simulink model "synchro_v3"  (R2020b)
settings: Solver=FixedStepAuto  StartTime=0.0  StopTime=2  FixedStep=Ts  RelTol=1e-3
values from neighbouring files (symbols this model uses):
  m = 5/100    (= 0.05)    [synchro_parameters_v1.m]
  Sbase = 1    [synchro_parameters_v1.m]
  Ts = 1/Fs    (= 0.0001)    [synchro_parameters_v1.m]
  Vbase = 1    [synchro_parameters_v1.m]
  w_droop = 10*2*pi    (= 62.8318530718)    [synchro_parameters_v1.m]
  w_pll = 10*2*pi    (= 62.8318530718)    [synchro_parameters_v1.m]
  w_tau = 1e3*2*pi    (= 6283.18530718)    [synchro_parameters_v1.m]
  Wbase = 2*pi*50    (= 314.159265359)    [synchro_parameters_v1.m]
  Ybase = 1/Zbase    (= 1)    [synchro_parameters_v1.m]
  Zbase = Vbase/Ibase    (= 1)    [synchro_parameters_v1.m]
undefined symbols (not defined in the file or in its folder): DiscIntNeverNeededParam
libraries: SimplexPS x69, powerlib x64
(part 2 of 2)

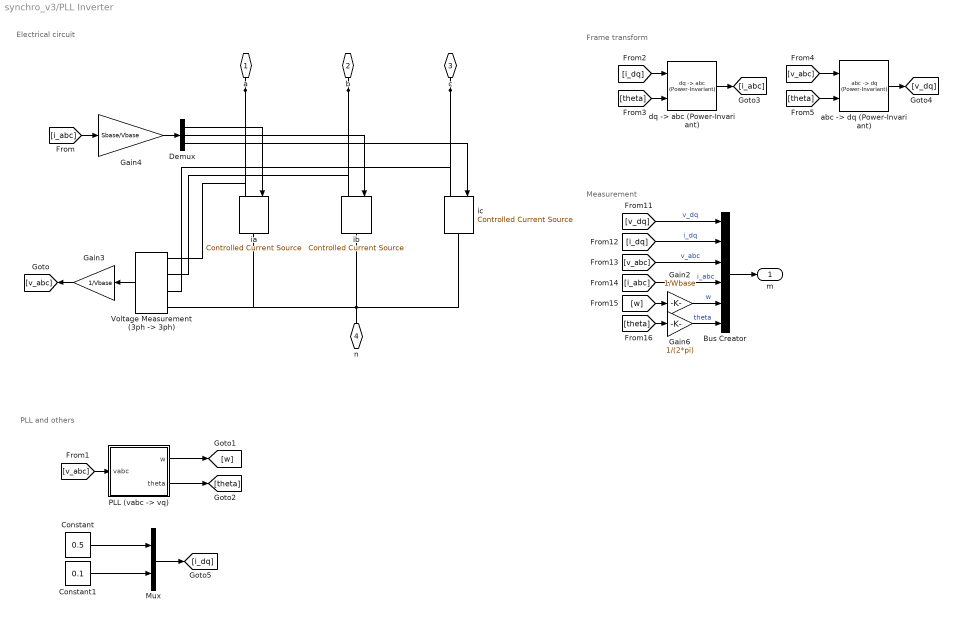
== system synchro_v3/PLL Inverter ==
  note: Measurement
  note: PLL and others
  note: Frame transform
  note: Electrical circuit
  Bus Creator : BusCreator  Inputs=6
  Constant : Constant  Value=0.5
  Constant1 : Constant  Value=0.1
  Demux : Demux  Outputs=3
  Gain2 : Gain  Gain=1/Wbase
  Gain3 : Gain  Gain=1/Vbase
  Gain4 : Gain  Gain=Sbase/Vbase
  Gain6 : Gain  Gain=1/(2*pi)
  Mux : Mux  Inputs=2
  "PLL (vabc -> vq)" : Subsystem  AncestorBlock=|  mask{Ts=Ts, Vbase=Vbase, Wbase=Wbase, w_pll=w_pll, w_tau=w_tau, theta0=0}
      | SimplexPS/PLL
      | (vabc -> vq)
      mask prompts: Ts "Ts (s), sampling period"; Vbase "Vbase (V), base voltage"; Wbase "Wbase (rad/s), base angular frequency"; w_pll "w_pll (rad/s), PLL bandwidth"; w_tau "w_tau (rad/s), low-pass filter bandwidth"; theta0 "theta0 (rad), initial angle"
  "Voltage Measurement (3ph -> 3ph)" : SimplexPS/Voltage Measurement (3ph -> 3ph)  SystemSampleTime=-1  VariantActivationTime=update diagram  Latency=0  AutoFrameSizeCalculation=off
      settings: SourceProductName=Simplex Power Systems
  "abc -> dq (Power-Invariant)" : SimplexPS/abc -> dq (Power-Invariant)  SystemSampleTime=-1  VariantActivationTime=update diagram  Latency=0  AutoFrameSizeCalculation=off
      settings: SourceProductName=Simplex Power Systems
  "dq -> abc (Power-Invariant)" : SimplexPS/dq -> abc (Power-Invariant)  SystemSampleTime=-1  VariantActivationTime=update diagram  Latency=0  AutoFrameSizeCalculation=off
      settings: SourceProductName=Simplex Power Systems
  ia : powerlib/Electrical Sources/Controlled Current Source  Initialize=on  Source_Type=AC  Amplitude=0  Phase=0  Frequency=0  Measurements=None
  ib : powerlib/Electrical Sources/Controlled Current Source  Initialize=on  Source_Type=AC  Amplitude=0  Phase=0  Frequency=0  Measurements=None
  ic : powerlib/Electrical Sources/Controlled Current Source  Initialize=on  Source_Type=AC  Amplitude=0  Phase=0  Frequency=0  Measurements=None
  a : PMIOPort  Side=Left
  b : PMIOPort  Port=2  Side=Left
  c : PMIOPort  Port=3  Side=Left
  n : PMIOPort  Port=4  Side=Left
  m : Outport
  wires:
  [v_dq] -> Bus Creator/1  "v_dq"
  [i_dq] -> Bus Creator/2  "i_dq"
  [v_abc] -> Bus Creator/3  "v_abc"
  [i_abc] -> Bus Creator/4  "i_abc"
  Bus Creator/1 -> m/1
  [w] -> Gain2/1
  Gain2/1 -> Bus Creator/5  "w"
  [i_abc] -> Gain4/1
  Gain4/1 -> Demux/1
  [theta] -> Gain6/1
  Gain6/1 -> Bus Creator/6  "theta"
  Demux/1 -> ia/1
  Demux/2 -> ib/1
  Demux/3 -> ic/1
  Gain3/1 -> [v_abc]
  [v_abc] -> "PLL (vabc -> vq)"/1(vabc)
  "PLL (vabc -> vq)"/1(w) -> [w]
  "PLL (vabc -> vq)"/2(theta) -> [theta]
  "Voltage Measurement (3ph -> 3ph)"/1 -> Gain3/1
  "dq -> abc (Power-Invariant)"/1 -> [i_abc]
  [i_dq] -> "dq -> abc (Power-Invariant)"/1
  [theta] -> "dq -> abc (Power-Invariant)"/2
  [v_abc] -> "abc -> dq (Power-Invariant)"/1
  [theta] -> "abc -> dq (Power-Invariant)"/2
  "abc -> dq (Power-Invariant)"/1 -> [v_dq]
  Constant/1 -> Mux/1
  Constant1/1 -> Mux/2
  Mux/1 -> [i_dq]
  connections:
  a/RConn1 -- "Voltage Measurement (3ph -> 3ph)"/LConn1 -- ia/LConn1
  ib/RConn1 -- ic/RConn1 -- n/RConn1 -- "Voltage Measurement (3ph -> 3ph)"/LConn4 -- ia/RConn1
  b/RConn1 -- "Voltage Measurement (3ph -> 3ph)"/LConn2 -- ib/LConn1
  c/RConn1 -- "Voltage Measurement (3ph -> 3ph)"/LConn3 -- ic/LConn1

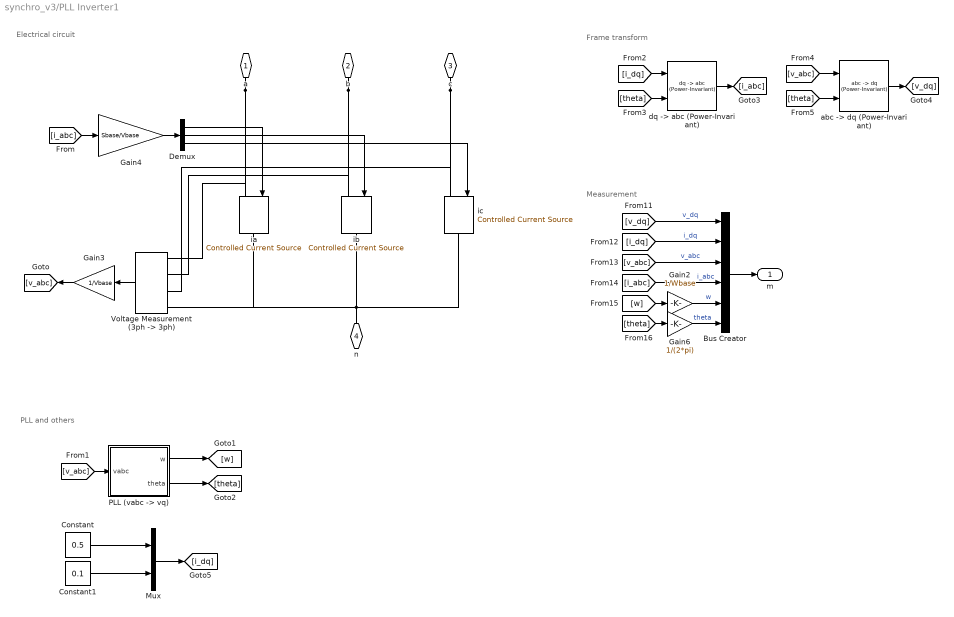
== system synchro_v3/PLL Inverter1 ==
  note: Measurement
  note: PLL and others
  note: Frame transform
  note: Electrical circuit
  Bus Creator : BusCreator  Inputs=6
  Constant : Constant  Value=0.5
  Constant1 : Constant  Value=0.1
  Demux : Demux  Outputs=3
  Gain2 : Gain  Gain=1/Wbase
  Gain3 : Gain  Gain=1/Vbase
  Gain4 : Gain  Gain=Sbase/Vbase
  Gain6 : Gain  Gain=1/(2*pi)
  Mux : Mux  Inputs=2
  "PLL (vabc -> vq)" : Subsystem  AncestorBlock=|  mask{Ts=Ts, Vbase=Vbase, Wbase=Wbase, w_pll=w_pll, w_tau=w_tau, theta0=0}
      | SimplexPS/PLL
      | (vabc -> vq)
      mask prompts: Ts "Ts (s), sampling period"; Vbase "Vbase (V), base voltage"; Wbase "Wbase (rad/s), base angular frequency"; w_pll "w_pll (rad/s), PLL bandwidth"; w_tau "w_tau (rad/s), low-pass filter bandwidth"; theta0 "theta0 (rad), initial angle"
  "Voltage Measurement (3ph -> 3ph)" : SimplexPS/Voltage Measurement (3ph -> 3ph)  SystemSampleTime=-1  VariantActivationTime=update diagram  Latency=0  AutoFrameSizeCalculation=off
      settings: SourceProductName=Simplex Power Systems
  "abc -> dq (Power-Invariant)" : SimplexPS/abc -> dq (Power-Invariant)  SystemSampleTime=-1  VariantActivationTime=update diagram  Latency=0  AutoFrameSizeCalculation=off
      settings: SourceProductName=Simplex Power Systems
  "dq -> abc (Power-Invariant)" : SimplexPS/dq -> abc (Power-Invariant)  SystemSampleTime=-1  VariantActivationTime=update diagram  Latency=0  AutoFrameSizeCalculation=off
      settings: SourceProductName=Simplex Power Systems
  ia : powerlib/Electrical Sources/Controlled Current Source  Initialize=on  Source_Type=AC  Amplitude=0  Phase=0  Frequency=0  Measurements=None
  ib : powerlib/Electrical Sources/Controlled Current Source  Initialize=on  Source_Type=AC  Amplitude=0  Phase=0  Frequency=0  Measurements=None
  ic : powerlib/Electrical Sources/Controlled Current Source  Initialize=on  Source_Type=AC  Amplitude=0  Phase=0  Frequency=0  Measurements=None
  a : PMIOPort  Side=Left
  b : PMIOPort  Port=2  Side=Left
  c : PMIOPort  Port=3  Side=Left
  n : PMIOPort  Port=4  Side=Left
  m : Outport
  wires:
  [v_dq] -> Bus Creator/1  "v_dq"
  [i_dq] -> Bus Creator/2  "i_dq"
  [v_abc] -> Bus Creator/3  "v_abc"
  [i_abc] -> Bus Creator/4  "i_abc"
  Bus Creator/1 -> m/1
  [w] -> Gain2/1
  Gain2/1 -> Bus Creator/5  "w"
  [i_abc] -> Gain4/1
  Gain4/1 -> Demux/1
  [theta] -> Gain6/1
  Gain6/1 -> Bus Creator/6  "theta"
  Demux/1 -> ia/1
  Demux/2 -> ib/1
  Demux/3 -> ic/1
  Gain3/1 -> [v_abc]
  [v_abc] -> "PLL (vabc -> vq)"/1(vabc)
  "PLL (vabc -> vq)"/1(w) -> [w]
  "PLL (vabc -> vq)"/2(theta) -> [theta]
  "Voltage Measurement (3ph -> 3ph)"/1 -> Gain3/1
  "dq -> abc (Power-Invariant)"/1 -> [i_abc]
  [i_dq] -> "dq -> abc (Power-Invariant)"/1
  [theta] -> "dq -> abc (Power-Invariant)"/2
  [v_abc] -> "abc -> dq (Power-Invariant)"/1
  [theta] -> "abc -> dq (Power-Invariant)"/2
  "abc -> dq (Power-Invariant)"/1 -> [v_dq]
  Constant/1 -> Mux/1
  Constant1/1 -> Mux/2
  Mux/1 -> [i_dq]
  connections:
  a/RConn1 -- ia/LConn1 -- "Voltage Measurement (3ph -> 3ph)"/LConn1
  ib/RConn1 -- ic/RConn1 -- n/RConn1 -- ia/RConn1 -- "Voltage Measurement (3ph -> 3ph)"/LConn4
  b/RConn1 -- ib/LConn1 -- "Voltage Measurement (3ph -> 3ph)"/LConn2
  c/RConn1 -- ic/LConn1 -- "Voltage Measurement (3ph -> 3ph)"/LConn3

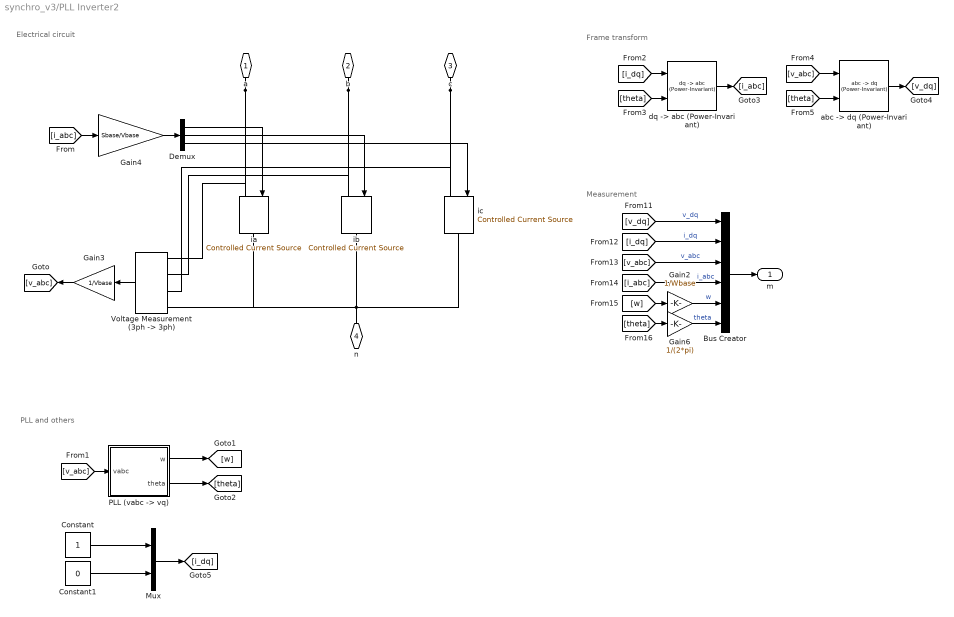
== system synchro_v3/PLL Inverter2 ==
  note: Measurement
  note: PLL and others
  note: Frame transform
  note: Electrical circuit
  Bus Creator : BusCreator  Inputs=6
  Constant : Constant
  Constant1 : Constant  Value=0
  Demux : Demux  Outputs=3
  Gain2 : Gain  Gain=1/Wbase
  Gain3 : Gain  Gain=1/Vbase
  Gain4 : Gain  Gain=Sbase/Vbase
  Gain6 : Gain  Gain=1/(2*pi)
  Mux : Mux  Inputs=2
  "PLL (vabc -> vq)" : Subsystem  AncestorBlock=|  mask{Ts=Ts, Vbase=Vbase, Wbase=Wbase, w_pll=w_pll, w_tau=w_tau, theta0=0}
      | SimplexPS/PLL
      | (vabc -> vq)
      mask prompts: Ts "Ts (s), sampling period"; Vbase "Vbase (V), base voltage"; Wbase "Wbase (rad/s), base angular frequency"; w_pll "w_pll (rad/s), PLL bandwidth"; w_tau "w_tau (rad/s), low-pass filter bandwidth"; theta0 "theta0 (rad), initial angle"
  "Voltage Measurement (3ph -> 3ph)" : SimplexPS/Voltage Measurement (3ph -> 3ph)  SystemSampleTime=-1  VariantActivationTime=update diagram  Latency=0  AutoFrameSizeCalculation=off
      settings: SourceProductName=Simplex Power Systems
  "abc -> dq (Power-Invariant)" : SimplexPS/abc -> dq (Power-Invariant)  SystemSampleTime=-1  VariantActivationTime=update diagram  Latency=0  AutoFrameSizeCalculation=off
      settings: SourceProductName=Simplex Power Systems
  "dq -> abc (Power-Invariant)" : SimplexPS/dq -> abc (Power-Invariant)  SystemSampleTime=-1  VariantActivationTime=update diagram  Latency=0  AutoFrameSizeCalculation=off
      settings: SourceProductName=Simplex Power Systems
  ia : powerlib/Electrical Sources/Controlled Current Source  Initialize=on  Source_Type=AC  Amplitude=0  Phase=0  Frequency=0  Measurements=None
  ib : powerlib/Electrical Sources/Controlled Current Source  Initialize=on  Source_Type=AC  Amplitude=0  Phase=0  Frequency=0  Measurements=None
  ic : powerlib/Electrical Sources/Controlled Current Source  Initialize=on  Source_Type=AC  Amplitude=0  Phase=0  Frequency=0  Measurements=None
  a : PMIOPort  Side=Left
  b : PMIOPort  Port=2  Side=Left
  c : PMIOPort  Port=3  Side=Left
  n : PMIOPort  Port=4  Side=Left
  m : Outport
  wires:
  [v_dq] -> Bus Creator/1  "v_dq"
  [i_dq] -> Bus Creator/2  "i_dq"
  [v_abc] -> Bus Creator/3  "v_abc"
  [i_abc] -> Bus Creator/4  "i_abc"
  Bus Creator/1 -> m/1
  [w] -> Gain2/1
  Gain2/1 -> Bus Creator/5  "w"
  [i_abc] -> Gain4/1
  Gain4/1 -> Demux/1
  [theta] -> Gain6/1
  Gain6/1 -> Bus Creator/6  "theta"
  Demux/1 -> ia/1
  Demux/2 -> ib/1
  Demux/3 -> ic/1
  Gain3/1 -> [v_abc]
  [v_abc] -> "PLL (vabc -> vq)"/1(vabc)
  "PLL (vabc -> vq)"/1(w) -> [w]
  "PLL (vabc -> vq)"/2(theta) -> [theta]
  "Voltage Measurement (3ph -> 3ph)"/1 -> Gain3/1
  "dq -> abc (Power-Invariant)"/1 -> [i_abc]
  [i_dq] -> "dq -> abc (Power-Invariant)"/1
  [theta] -> "dq -> abc (Power-Invariant)"/2
  [v_abc] -> "abc -> dq (Power-Invariant)"/1
  [theta] -> "abc -> dq (Power-Invariant)"/2
  "abc -> dq (Power-Invariant)"/1 -> [v_dq]
  Constant/1 -> Mux/1
  Constant1/1 -> Mux/2
  Mux/1 -> [i_dq]
  connections:
  a/RConn1 -- ia/LConn1 -- "Voltage Measurement (3ph -> 3ph)"/LConn1
  ib/RConn1 -- ic/RConn1 -- n/RConn1 -- ia/RConn1 -- "Voltage Measurement (3ph -> 3ph)"/LConn4
  b/RConn1 -- ib/LConn1 -- "Voltage Measurement (3ph -> 3ph)"/LConn2
  c/RConn1 -- ic/LConn1 -- "Voltage Measurement (3ph -> 3ph)"/LConn3

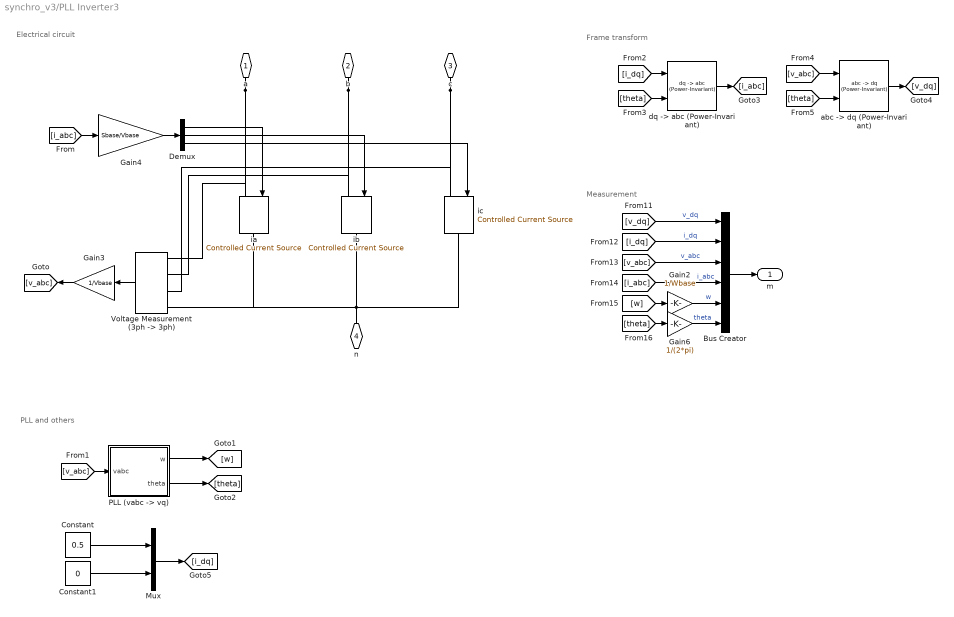
== system synchro_v3/PLL Inverter3 ==
  note: Measurement
  note: PLL and others
  note: Frame transform
  note: Electrical circuit
  Bus Creator : BusCreator  Inputs=6
  Constant : Constant  Value=0.5
  Constant1 : Constant  Value=0
  Demux : Demux  Outputs=3
  Gain2 : Gain  Gain=1/Wbase
  Gain3 : Gain  Gain=1/Vbase
  Gain4 : Gain  Gain=Sbase/Vbase
  Gain6 : Gain  Gain=1/(2*pi)
  Mux : Mux  Inputs=2
  "PLL (vabc -> vq)" : Subsystem  AncestorBlock=|  mask{Ts=Ts, Vbase=Vbase, Wbase=Wbase, w_pll=w_pll, w_tau=w_tau, theta0=0}
      | SimplexPS/PLL
      | (vabc -> vq)
      mask prompts: Ts "Ts (s), sampling period"; Vbase "Vbase (V), base voltage"; Wbase "Wbase (rad/s), base angular frequency"; w_pll "w_pll (rad/s), PLL bandwidth"; w_tau "w_tau (rad/s), low-pass filter bandwidth"; theta0 "theta0 (rad), initial angle"
  "Voltage Measurement (3ph -> 3ph)" : SimplexPS/Voltage Measurement (3ph -> 3ph)  SystemSampleTime=-1  VariantActivationTime=update diagram  Latency=0  AutoFrameSizeCalculation=off
      settings: SourceProductName=Simplex Power Systems
  "abc -> dq (Power-Invariant)" : SimplexPS/abc -> dq (Power-Invariant)  SystemSampleTime=-1  VariantActivationTime=update diagram  Latency=0  AutoFrameSizeCalculation=off
      settings: SourceProductName=Simplex Power Systems
  "dq -> abc (Power-Invariant)" : SimplexPS/dq -> abc (Power-Invariant)  SystemSampleTime=-1  VariantActivationTime=update diagram  Latency=0  AutoFrameSizeCalculation=off
      settings: SourceProductName=Simplex Power Systems
  ia : powerlib/Electrical Sources/Controlled Current Source  Initialize=on  Source_Type=AC  Amplitude=0  Phase=0  Frequency=0  Measurements=None
  ib : powerlib/Electrical Sources/Controlled Current Source  Initialize=on  Source_Type=AC  Amplitude=0  Phase=0  Frequency=0  Measurements=None
  ic : powerlib/Electrical Sources/Controlled Current Source  Initialize=on  Source_Type=AC  Amplitude=0  Phase=0  Frequency=0  Measurements=None
  a : PMIOPort  Side=Left
  b : PMIOPort  Port=2  Side=Left
  c : PMIOPort  Port=3  Side=Left
  n : PMIOPort  Port=4  Side=Left
  m : Outport
  wires:
  [v_dq] -> Bus Creator/1  "v_dq"
  [i_dq] -> Bus Creator/2  "i_dq"
  [v_abc] -> Bus Creator/3  "v_abc"
  [i_abc] -> Bus Creator/4  "i_abc"
  Bus Creator/1 -> m/1
  [w] -> Gain2/1
  Gain2/1 -> Bus Creator/5  "w"
  [i_abc] -> Gain4/1
  Gain4/1 -> Demux/1
  [theta] -> Gain6/1
  Gain6/1 -> Bus Creator/6  "theta"
  Demux/1 -> ia/1
  Demux/2 -> ib/1
  Demux/3 -> ic/1
  Gain3/1 -> [v_abc]
  [v_abc] -> "PLL (vabc -> vq)"/1(vabc)
  "PLL (vabc -> vq)"/1(w) -> [w]
  "PLL (vabc -> vq)"/2(theta) -> [theta]
  "Voltage Measurement (3ph -> 3ph)"/1 -> Gain3/1
  "dq -> abc (Power-Invariant)"/1 -> [i_abc]
  [i_dq] -> "dq -> abc (Power-Invariant)"/1
  [theta] -> "dq -> abc (Power-Invariant)"/2
  [v_abc] -> "abc -> dq (Power-Invariant)"/1
  [theta] -> "abc -> dq (Power-Invariant)"/2
  "abc -> dq (Power-Invariant)"/1 -> [v_dq]
  Constant/1 -> Mux/1
  Constant1/1 -> Mux/2
  Mux/1 -> [i_dq]
  connections:
  a/RConn1 -- ia/LConn1 -- "Voltage Measurement (3ph -> 3ph)"/LConn1
  ib/RConn1 -- ic/RConn1 -- n/RConn1 -- ia/RConn1 -- "Voltage Measurement (3ph -> 3ph)"/LConn4
  b/RConn1 -- ib/LConn1 -- "Voltage Measurement (3ph -> 3ph)"/LConn2
  c/RConn1 -- ic/LConn1 -- "Voltage Measurement (3ph -> 3ph)"/LConn3

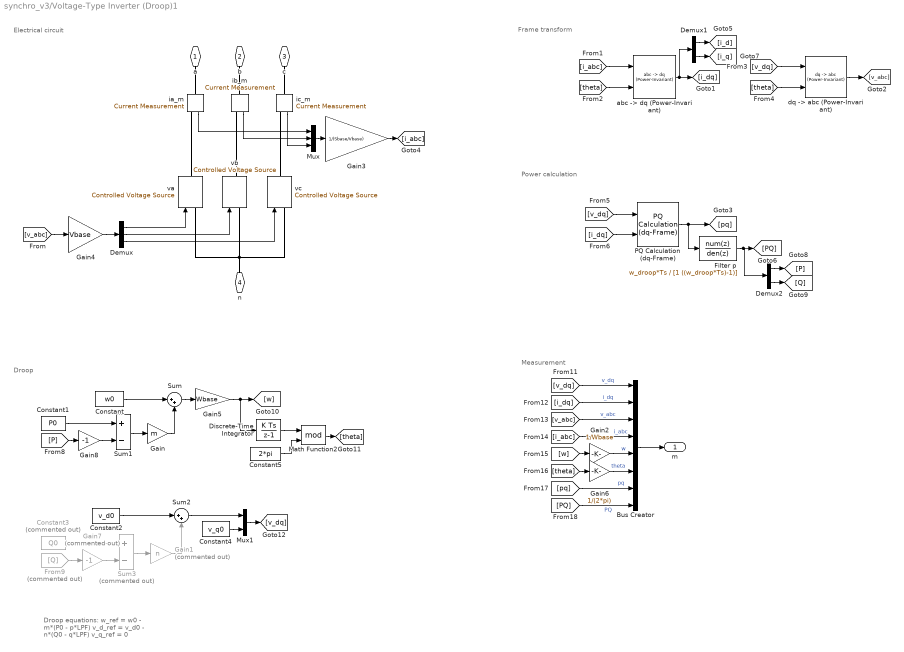
== system synchro_v3/Voltage-Type Inverter (Droop)1 ==
  note: Droop equations:
      | w_ref = w0 - m*(P0 - p*LPF)
      | v_d_ref = v_d0 - n*(Q0 - q*LPF)
      | v_q_ref = 0
  note: Measurement
  note: Droop
  note: Power calculation
  note: Frame transform
  note: Electrical circuit
  Bus Creator : BusCreator  Inputs=8
  Constant : Constant  Value=w0
  Constant1 : Constant  Value=P0
  Constant2 : Constant  Value=v_d0
  Constant3 : Constant  Commented=on  Value=Q0
  Constant4 : Constant  Value=v_q0
  Constant5 : Constant  Value=2*pi
  Demux : Demux  Outputs=3
  Demux1 : Demux  Outputs=2
  Demux2 : Demux  Outputs=2
  Discrete-Time Integrator : DiscreteIntegrator  SampleTime=Ts  ICPrevOutput=DiscIntNeverNeededParam  ICPrevScaledInput=DiscIntNeverNeededParam
  Filter p : DiscreteTransferFcn  Numerator=w_droop*Ts  Denominator=[1 ((w_droop*Ts)-1)]  SampleTime=Ts
  From9 : From  Commented=on  GotoTag=Q
  Gain : Gain  Gain=m
  Gain1 : Gain  Commented=on  Gain=n
  Gain2 : Gain  Gain=1/Wbase
  Gain3 : Gain  Gain=1/(Sbase/Vbase)
  Gain4 : Gain  Gain=Vbase
  Gain5 : Gain  Gain=Wbase
  Gain6 : Gain  Gain=1/(2*pi)
  Gain7 : Gain  Commented=on  Gain=-1
  Gain8 : Gain  Gain=-1
  Math Function2 : Math  Operator=mod  SignedPower=on  SaturateOnIntegerOverflow=on
  Mux : Mux  Inputs=3
  Mux1 : Mux  Inputs=2
  PQ Calculation (dq-Frame) : SimplexPS/PQ Calculation (dq-Frame)  SystemSampleTime=-1  VariantActivationTime=update diagram  Latency=0  AutoFrameSizeCalculation=off
      settings: SourceProductName=Simplex Power Systems
  Sum : Sum  Inputs=|++
  Sum1 : Sum  Inputs=+-
  Sum2 : Sum  Inputs=|++
  Sum3 : Sum  Commented=on  Inputs=+-
  "abc -> dq (Power-Invariant)" : SimplexPS/abc -> dq (Power-Invariant)  SystemSampleTime=-1  VariantActivationTime=update diagram  Latency=0  AutoFrameSizeCalculation=off
      settings: SourceProductName=Simplex Power Systems
  "dq -> abc (Power-Invariant)" : SimplexPS/dq -> abc (Power-Invariant)  SystemSampleTime=-1  VariantActivationTime=update diagram  Latency=0  AutoFrameSizeCalculation=off
      settings: SourceProductName=Simplex Power Systems
  ia_m : powerlib/Measurements/Current Measurement  PhasorSimulation=off  OutputType=Complex  PSBequivalent=0
  ib_m : powerlib/Measurements/Current Measurement  PhasorSimulation=off  OutputType=Complex  PSBequivalent=0
  ic_m : powerlib/Measurements/Current Measurement  PhasorSimulation=off  OutputType=Complex  PSBequivalent=0
  va : powerlib/Electrical Sources/Controlled Voltage Source  Initialize=on  Source_Type=AC  Amplitude=0  Phase=0  Frequency=0  Measurements=None
  vb : powerlib/Electrical Sources/Controlled Voltage Source  Initialize=on  Source_Type=AC  Amplitude=0  Phase=0  Frequency=0  Measurements=None
  vc : powerlib/Electrical Sources/Controlled Voltage Source  Initialize=on  Source_Type=AC  Amplitude=0  Phase=0  Frequency=0  Measurements=None
  a : PMIOPort  Side=Left
  b : PMIOPort  Port=2  Side=Left
  c : PMIOPort  Port=3  Side=Left
  n : PMIOPort  Port=4  Side=Left
  m : Outport
  wires:
  ic_m/1 -> Mux/3
  ia_m/1 -> Mux/1
  ib_m/1 -> Mux/2
  Demux/1 -> va/1
  Demux/2 -> vb/1
  Demux/3 -> vc/1
  [i_abc] -> "abc -> dq (Power-Invariant)"/1
  [theta] -> "abc -> dq (Power-Invariant)"/2
  "abc -> dq (Power-Invariant)"/1 -> Demux1/1, [i_dq]
  [v_dq] -> "dq -> abc (Power-Invariant)"/1
  [theta] -> "dq -> abc (Power-Invariant)"/2
  "dq -> abc (Power-Invariant)"/1 -> [v_abc]
  [v_dq] -> PQ Calculation (dq-Frame)/1
  [i_dq] -> PQ Calculation (dq-Frame)/2
  PQ Calculation (dq-Frame)/1 -> Filter p/1, [pq]
  Constant/1 -> Sum/1
  Constant1/1 -> Sum1/1
  Demux2/1 -> [P]
  Demux2/2 -> [Q]
  Gain/1 -> Sum/2
  Sum/1 -> Gain5/1
  Constant2/1 -> Sum2/1
  Sum3/1 -> Gain1/1
  Constant3/1 -> Sum3/1
  Gain1/1 -> Sum2/2
  Sum2/1 -> Mux1/1
  Constant4/1 -> Mux1/2
  Mux1/1 -> [v_dq]
  [v_dq] -> Bus Creator/1  "v_dq"
  [i_dq] -> Bus Creator/2  "i_dq"
  [v_abc] -> Bus Creator/3  "v_abc"
  [i_abc] -> Bus Creator/4  "i_abc"
  [pq] -> Bus Creator/7  "pq"
  [PQ] -> Bus Creator/8  "PQ"
  Bus Creator/1 -> m/1
  [w] -> Gain2/1
  Gain2/1 -> Bus Creator/5  "w"
  Mux/1 -> Gain3/1
  Gain3/1 -> [i_abc]
  [v_abc] -> Gain4/1
  Gain4/1 -> Demux/1
  Gain5/1 -> Discrete-Time Integrator/1, [w]
  Discrete-Time Integrator/1 -> Math Function2/1
  Math Function2/1 -> [theta]
  Constant5/1 -> Math Function2/2
  [theta] -> Gain6/1
  Gain6/1 -> Bus Creator/6  "theta"
  From9/1 -> Gain7/1
  Gain7/1 -> Sum3/2
  [P] -> Gain8/1
  Gain8/1 -> Sum1/2
  Demux1/2 -> [i_q]
  Demux1/1 -> [i_d]
  Sum1/1 -> Gain/1
  Filter p/1 -> Demux2/1, [PQ]
  connections:
  ia_m/RConn1 -- va/RConn1
  ia_m/LConn1 -- a/RConn1
  ib_m/RConn1 -- vb/RConn1
  ic_m/RConn1 -- vc/RConn1
  va/LConn1 -- vb/LConn1 -- vc/LConn1 -- n/RConn1
  ib_m/LConn1 -- b/RConn1
  ic_m/LConn1 -- c/RConn1

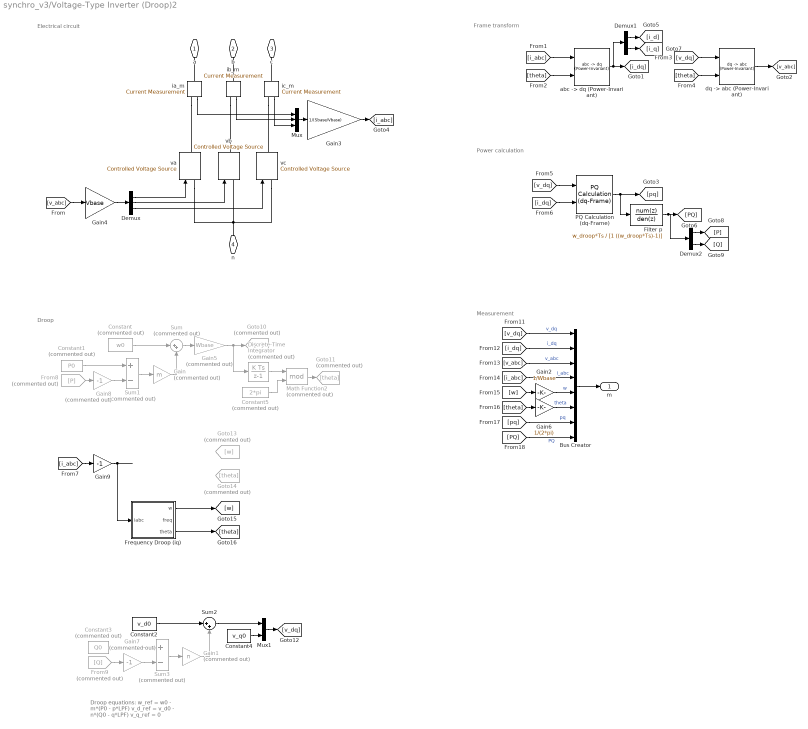
== system synchro_v3/Voltage-Type Inverter (Droop)2 ==
  note: Droop equations:
      | w_ref = w0 - m*(P0 - p*LPF)
      | v_d_ref = v_d0 - n*(Q0 - q*LPF)
      | v_q_ref = 0
  note: Measurement
  note: Droop
  note: Power calculation
  note: Frame transform
  note: Electrical circuit
  Bus Creator : BusCreator  Inputs=8
  Constant : Constant  Commented=on  Value=w0
  Constant1 : Constant  Commented=on  Value=P0
  Constant2 : Constant  Value=v_d0
  Constant3 : Constant  Commented=on  Value=Q0
  Constant4 : Constant  Value=v_q0
  Constant5 : Constant  Commented=on  Value=2*pi
  Demux : Demux  Outputs=3
  Demux1 : Demux  Outputs=2
  Demux2 : Demux  Outputs=2
  Discrete-Time Integrator : DiscreteIntegrator  Commented=on  SampleTime=Ts  ICPrevOutput=DiscIntNeverNeededParam  ICPrevScaledInput=DiscIntNeverNeededParam
  Filter p : DiscreteTransferFcn  Numerator=w_droop*Ts  Denominator=[1 ((w_droop*Ts)-1)]  SampleTime=Ts
  Frequency Droop (iq) : Subsystem  AncestorBlock=SimplexPS/Frequency Droop (iq)  mask{Ts=Ts, Sbase=Sbase, Vbase=Vbase, Wbase=Wbase, m=m, w_tau=w_droop, theta0=0, P0=0, W0=1}
      mask prompts: Ts "Ts (s), samping period"; Sbase "Sbase (VA), base power"; Vbase "Vbase (V), base voltage"; Wbase "Wbase (rad/s), base angular frequency"; m "m (pu), droop gain"; w_tau "w_tau (rad/s), low-pass filter bandwidth"; theta0 "theta0 (rad), initial angle"; P0 "P0 (pu), power setting point"; W0 "W0 (pu), frequency setting point"
  From8 : From  Commented=on  GotoTag=P
  From9 : From  Commented=on  GotoTag=Q
  Gain : Gain  Commented=on  Gain=m
  Gain1 : Gain  Commented=on  Gain=n
  Gain2 : Gain  Gain=1/Wbase
  Gain3 : Gain  Gain=1/(Sbase/Vbase)
  Gain4 : Gain  Gain=Vbase
  Gain5 : Gain  Commented=on  Gain=Wbase
  Gain6 : Gain  Gain=1/(2*pi)
  Gain7 : Gain  Commented=on  Gain=-1
  Gain8 : Gain  Commented=on  Gain=-1
  Gain9 : Gain  Gain=-1
  Goto10 : Goto  Commented=on  GotoTag=w
  Goto11 : Goto  Commented=on  GotoTag=theta
  Goto13 : Goto  Commented=on  GotoTag=w
  Goto14 : Goto  Commented=on  GotoTag=theta
  Math Function2 : Math  Commented=on  Operator=mod  SignedPower=on  SaturateOnIntegerOverflow=on
  Mux : Mux  Inputs=3
  Mux1 : Mux  Inputs=2
  PQ Calculation (dq-Frame) : SimplexPS/PQ Calculation (dq-Frame)  SystemSampleTime=-1  VariantActivationTime=update diagram  Latency=0  AutoFrameSizeCalculation=off
      settings: SourceProductName=Simplex Power Systems
  Sum : Sum  Commented=on  Inputs=|++
  Sum1 : Sum  Commented=on  Inputs=+-
  Sum2 : Sum  Inputs=|++
  Sum3 : Sum  Commented=on  Inputs=+-
  "abc -> dq (Power-Invariant)" : SimplexPS/abc -> dq (Power-Invariant)  SystemSampleTime=-1  VariantActivationTime=update diagram  Latency=0  AutoFrameSizeCalculation=off
      settings: SourceProductName=Simplex Power Systems
  "dq -> abc (Power-Invariant)" : SimplexPS/dq -> abc (Power-Invariant)  SystemSampleTime=-1  VariantActivationTime=update diagram  Latency=0  AutoFrameSizeCalculation=off
      settings: SourceProductName=Simplex Power Systems
  ia_m : powerlib/Measurements/Current Measurement  PhasorSimulation=off  OutputType=Complex  PSBequivalent=0
  ib_m : powerlib/Measurements/Current Measurement  PhasorSimulation=off  OutputType=Complex  PSBequivalent=0
  ic_m : powerlib/Measurements/Current Measurement  PhasorSimulation=off  OutputType=Complex  PSBequivalent=0
  va : powerlib/Electrical Sources/Controlled Voltage Source  Initialize=on  Source_Type=AC  Amplitude=0  Phase=0  Frequency=0  Measurements=None
  vb : powerlib/Electrical Sources/Controlled Voltage Source  Initialize=on  Source_Type=AC  Amplitude=0  Phase=0  Frequency=0  Measurements=None
  vc : powerlib/Electrical Sources/Controlled Voltage Source  Initialize=on  Source_Type=AC  Amplitude=0  Phase=0  Frequency=0  Measurements=None
  a : PMIOPort  Side=Left
  b : PMIOPort  Port=2  Side=Left
  c : PMIOPort  Port=3  Side=Left
  n : PMIOPort  Port=4  Side=Left
  m : Outport
  wires:
  ic_m/1 -> Mux/3
  ia_m/1 -> Mux/1
  ib_m/1 -> Mux/2
  Demux/1 -> va/1
  Demux/2 -> vb/1
  Demux/3 -> vc/1
  [i_abc] -> "abc -> dq (Power-Invariant)"/1
  [theta] -> "abc -> dq (Power-Invariant)"/2
  "abc -> dq (Power-Invariant)"/1 -> Demux1/1, [i_dq]
  [v_dq] -> "dq -> abc (Power-Invariant)"/1
  [theta] -> "dq -> abc (Power-Invariant)"/2
  "dq -> abc (Power-Invariant)"/1 -> [v_abc]
  [v_dq] -> PQ Calculation (dq-Frame)/1
  [i_dq] -> PQ Calculation (dq-Frame)/2
  PQ Calculation (dq-Frame)/1 -> Filter p/1, [pq]
  Constant/1 -> Sum/1
  Constant1/1 -> Sum1/1
  Demux2/1 -> [P]
  Demux2/2 -> [Q]
  Gain/1 -> Sum/2
  Sum/1 -> Gain5/1
  Constant2/1 -> Sum2/1
  Sum3/1 -> Gain1/1
  Constant3/1 -> Sum3/1
  Gain1/1 -> Sum2/2
  Sum2/1 -> Mux1/1
  Constant4/1 -> Mux1/2
  Mux1/1 -> [v_dq]
  [v_dq] -> Bus Creator/1  "v_dq"
  [i_dq] -> Bus Creator/2  "i_dq"
  [v_abc] -> Bus Creator/3  "v_abc"
  [i_abc] -> Bus Creator/4  "i_abc"
  [pq] -> Bus Creator/7  "pq"
  [PQ] -> Bus Creator/8  "PQ"
  Bus Creator/1 -> m/1
  [w] -> Gain2/1
  Gain2/1 -> Bus Creator/5  "w"
  Mux/1 -> Gain3/1
  Gain3/1 -> [i_abc]
  [v_abc] -> Gain4/1
  Gain4/1 -> Demux/1
  Gain5/1 -> Discrete-Time Integrator/1, Goto10/1
  Discrete-Time Integrator/1 -> Math Function2/1
  Math Function2/1 -> Goto11/1
  Constant5/1 -> Math Function2/2
  [theta] -> Gain6/1
  Gain6/1 -> Bus Creator/6  "theta"
  From9/1 -> Gain7/1
  Gain7/1 -> Sum3/2
  From8/1 -> Gain8/1
  Gain8/1 -> Sum1/2
  Demux1/2 -> [i_q]
  Demux1/1 -> [i_d]
  Sum1/1 -> Gain/1
  Filter p/1 -> Demux2/1, [PQ]
  ? -> Goto13/1
  ? -> Goto14/1
  [i_abc] -> Gain9/1
  Gain9/1 -> Frequency Droop (iq)/1(iabc)
  Frequency Droop (iq)/3(theta) -> [theta]
  Frequency Droop (iq)/1(w) -> [w]
  connections:
  ia_m/RConn1 -- va/RConn1
  ia_m/LConn1 -- a/RConn1
  ib_m/RConn1 -- vb/RConn1
  ic_m/RConn1 -- vc/RConn1
  va/LConn1 -- vb/LConn1 -- vc/LConn1 -- n/RConn1
  ib_m/LConn1 -- b/RConn1
  ic_m/LConn1 -- c/RConn1

== system synchro_v3/Droop Inverter1/Frequency Droop (iabc -> id) ==
  note: Measurement
  note: Notes: The current reference should be in source convention.
  iabc : Inport
  1st Order LPF (Trapezoidal) : SimplexPS/1st Order LPF (Trapezoidal)  Ts=Ts  wc=w_tau
      settings: SourceProductName=Simplex Power Systems
  Constant : Constant  Value=w0
  Constant2 : Constant  Value=theta0
  Constant4 : Constant  Value=2*pi
  Constant6 : Constant  Value=i0
  Demux1 : Demux  Outputs=2
  Discrete-Time Integrator : DiscreteIntegrator  IntegratorMethod=Integration: Trapezoidal  SampleTime=Ts  ICPrevOutput=DiscIntNeverNeededParam  ICPrevScaledInput=DiscIntNeverNeededParam
  Gain1 : Gain  Gain=1/(Sbase/Vbase)
  Gain2 : Gain  Gain=m
  Gain3 : Gain  Gain=Wbase
  Gain4 : Gain  Gain=1/Wbase
  Gain5 : Gain  Gain=1/pi
  Math Function1 : Math  Operator=mod  SignedPower=on  SaturateOnIntegerOverflow=on
  Mux : Mux  Inputs=2
  Scope : Scope  NumInputPorts=4
  Sum : Sum
  Sum1 : Sum
  Sum2 : Sum  Inputs=+-
  "abc -> dq (Power-Invariant)" : SimplexPS/abc -> dq (Power-Invariant)  SystemSampleTime=-1  VariantActivationTime=update diagram  Latency=0  AutoFrameSizeCalculation=off
      settings: SourceProductName=Simplex Power Systems
  w : Outport
  theta : Outport  Port=2
  wires:
  Gain4/1 -> Scope/3
  [w] -> Gain4/1  "w"
  Demux1/2 -> [iq]
  [theta] -> Mux/2  "theta"
  Mux/1 -> Gain5/1  "theta"
  [id] -> Scope/1  "id"
  [theta0] -> Mux/1  "theta"
  [iq] -> Scope/2  "iq"
  Gain5/1 -> Scope/4
  Demux1/1 -> [id], Gain1/1  "id"
  Gain3/1 -> Discrete-Time Integrator/1, w/1, [w]
  Sum/1 -> Gain3/1
  Sum2/1 -> Gain2/1
  Constant6/1 -> Sum2/1
  iabc/1 -> "abc -> dq (Power-Invariant)"/1
  Constant4/1 -> Math Function1/2
  "abc -> dq (Power-Invariant)"/1 -> Demux1/1
  Constant/1 -> Sum/2
  Gain1/1 -> 1st Order LPF (Trapezoidal)/1
  Discrete-Time Integrator/1 -> Sum1/1
  Gain2/1 -> Sum/1
  Math Function1/1 -> theta/1, [theta], "abc -> dq (Power-Invariant)"/2
  Constant2/1 -> [theta0], Sum1/2
  Sum1/1 -> Math Function1/1
  1st Order LPF (Trapezoidal)/1 -> Sum2/2

== system synchro_v3/PLL Inverter/PLL (vabc -> vq) ==
  note: Measurement
  note: Gpll
  vabc : Inport
  Constant1 : Constant
  Constant2 : Constant  Value=theta0
  Constant3 : Constant
  Constant4 : Constant  Value=2*pi
  Constant6 : Constant  Value=0
  Demux1 : Demux  Outputs=2
  Discrete PI : SimplexPS/Discrete PI  Kp=w_pll  Ki=w_pll^2/4/10  xmax=inf  xmin=-inf  Ts=Ts
      settings: SourceProductName=Simplex Power Systems
  Discrete-Time Integrator : DiscreteIntegrator  SampleTime=Ts  ICPrevOutput=DiscIntNeverNeededParam  ICPrevScaledInput=DiscIntNeverNeededParam
  Filter p : DiscreteTransferFcn  Numerator=w_tau*Ts  Denominator=[1 ((w_tau*Ts)-1)]  SampleTime=Ts
  Gain1 : Gain  Gain=Wbase
  Gain2 : Gain  Gain=1/Vbase
  Gain4 : Gain  Gain=1/Wbase
  Gain5 : Gain  Gain=1/pi
  Math Function1 : Math  Operator=mod  SignedPower=on  SaturateOnIntegerOverflow=on
  Mux : Mux  Inputs=2
  Scope : Scope  NumInputPorts=4
  Sum : Sum
  Sum1 : Sum
  "abc -> dq (Power-Invariant)" : SimplexPS/abc -> dq (Power-Invariant)  SystemSampleTime=-1  VariantActivationTime=update diagram  Latency=0  AutoFrameSizeCalculation=off
      settings: SourceProductName=Simplex Power Systems
  w : Outport
  theta : Outport  Port=2
  wires:
  vabc/1 -> "abc -> dq (Power-Invariant)"/1
  "abc -> dq (Power-Invariant)"/1 -> Demux1/1
  Constant4/1 -> Math Function1/2
  Gain2/1 -> Filter p/1
  Demux1/2 -> [vq], Gain2/1
  Constant6/1 -> Discrete PI/4, Discrete PI/3
  Constant1/1 -> Discrete PI/1
  Discrete PI/1 -> Sum/1
  Sum/1 -> [w], w/1, Discrete-Time Integrator/1
  Gain1/1 -> Sum/2
  Discrete-Time Integrator/1 -> Sum1/1
  Sum1/1 -> Math Function1/1
  Constant2/1 -> [theta0], Sum1/2
  Filter p/1 -> Discrete PI/2
  [vq] -> Scope/2  "vq"
  Mux/1 -> Gain5/1
  Gain4/1 -> Scope/3
  [w] -> Gain4/1  "w"
  [theta0] -> Mux/1  "theta0"
  [vd] -> Scope/1  "vd"
  Gain5/1 -> Scope/4
  [theta] -> Mux/2  "theta"
  Demux1/1 -> [vd]
  Constant3/1 -> Gain1/1
  Math Function1/1 -> "abc -> dq (Power-Invariant)"/2, [theta], theta/1

== system synchro_v3/PLL Inverter1/PLL (vabc -> vq) ==
  note: Measurement
  note: Gpll
  vabc : Inport
  Constant1 : Constant
  Constant2 : Constant  Value=theta0
  Constant3 : Constant
  Constant4 : Constant  Value=2*pi
  Constant6 : Constant  Value=0
  Demux1 : Demux  Outputs=2
  Discrete PI : SimplexPS/Discrete PI  Kp=w_pll  Ki=w_pll^2/4  xmax=inf  xmin=-inf  Ts=Ts
      settings: SourceProductName=Simplex Power Systems
  Discrete-Time Integrator : DiscreteIntegrator  SampleTime=Ts  ICPrevOutput=DiscIntNeverNeededParam  ICPrevScaledInput=DiscIntNeverNeededParam
  Filter p : DiscreteTransferFcn  Numerator=w_tau*Ts  Denominator=[1 ((w_tau*Ts)-1)]  SampleTime=Ts
  Gain1 : Gain  Gain=Wbase
  Gain2 : Gain  Gain=1/Vbase
  Gain4 : Gain  Gain=1/Wbase
  Gain5 : Gain  Gain=1/pi
  Math Function1 : Math  Operator=mod  SignedPower=on  SaturateOnIntegerOverflow=on
  Mux : Mux  Inputs=2
  Scope : Scope  NumInputPorts=4
  Sum : Sum
  Sum1 : Sum
  "abc -> dq (Power-Invariant)" : SimplexPS/abc -> dq (Power-Invariant)  SystemSampleTime=-1  VariantActivationTime=update diagram  Latency=0  AutoFrameSizeCalculation=off
      settings: SourceProductName=Simplex Power Systems
  w : Outport
  theta : Outport  Port=2
  wires:
  vabc/1 -> "abc -> dq (Power-Invariant)"/1
  "abc -> dq (Power-Invariant)"/1 -> Demux1/1
  Constant4/1 -> Math Function1/2
  Gain2/1 -> Filter p/1
  Demux1/2 -> [vq], Gain2/1
  Constant6/1 -> Discrete PI/4, Discrete PI/3
  Constant1/1 -> Discrete PI/1
  Discrete PI/1 -> Sum/1
  Sum/1 -> [w], w/1, Discrete-Time Integrator/1
  Gain1/1 -> Sum/2
  Discrete-Time Integrator/1 -> Sum1/1
  Sum1/1 -> Math Function1/1
  Constant2/1 -> [theta0], Sum1/2
  Filter p/1 -> Discrete PI/2
  [vq] -> Scope/2  "vq"
  Mux/1 -> Gain5/1
  Gain4/1 -> Scope/3
  [w] -> Gain4/1  "w"
  [theta0] -> Mux/1  "theta0"
  [vd] -> Scope/1  "vd"
  Gain5/1 -> Scope/4
  [theta] -> Mux/2  "theta"
  Demux1/1 -> [vd]
  Constant3/1 -> Gain1/1
  Math Function1/1 -> "abc -> dq (Power-Invariant)"/2, [theta], theta/1

== system synchro_v3/PLL Inverter2/PLL (vabc -> vq) ==
  note: Measurement
  note: Gpll
  vabc : Inport
  Constant1 : Constant
  Constant2 : Constant  Value=theta0
  Constant3 : Constant
  Constant4 : Constant  Value=2*pi
  Constant6 : Constant  Value=0
  Demux1 : Demux  Outputs=2
  Discrete PI : SimplexPS/Discrete PI  Kp=w_pll  Ki=w_pll^2/4  xmax=inf  xmin=-inf  Ts=Ts
      settings: SourceProductName=Simplex Power Systems
  Discrete-Time Integrator : DiscreteIntegrator  SampleTime=Ts  ICPrevOutput=DiscIntNeverNeededParam  ICPrevScaledInput=DiscIntNeverNeededParam
  Filter p : DiscreteTransferFcn  Numerator=w_tau*Ts  Denominator=[1 ((w_tau*Ts)-1)]  SampleTime=Ts
  Gain1 : Gain  Gain=Wbase
  Gain2 : Gain  Gain=1/Vbase
  Gain4 : Gain  Gain=1/Wbase
  Gain5 : Gain  Gain=1/pi
  Math Function1 : Math  Operator=mod  SignedPower=on  SaturateOnIntegerOverflow=on
  Mux : Mux  Inputs=2
  Scope : Scope  NumInputPorts=4
  Sum : Sum
  Sum1 : Sum
  "abc -> dq (Power-Invariant)" : SimplexPS/abc -> dq (Power-Invariant)  SystemSampleTime=-1  VariantActivationTime=update diagram  Latency=0  AutoFrameSizeCalculation=off
      settings: SourceProductName=Simplex Power Systems
  w : Outport
  theta : Outport  Port=2
  wires:
  vabc/1 -> "abc -> dq (Power-Invariant)"/1
  "abc -> dq (Power-Invariant)"/1 -> Demux1/1
  Constant4/1 -> Math Function1/2
  Gain2/1 -> Filter p/1
  Demux1/2 -> [vq], Gain2/1
  Constant6/1 -> Discrete PI/4, Discrete PI/3
  Constant1/1 -> Discrete PI/1
  Discrete PI/1 -> Sum/1
  Sum/1 -> [w], w/1, Discrete-Time Integrator/1
  Gain1/1 -> Sum/2
  Discrete-Time Integrator/1 -> Sum1/1
  Sum1/1 -> Math Function1/1
  Constant2/1 -> [theta0], Sum1/2
  Filter p/1 -> Discrete PI/2
  [vq] -> Scope/2  "vq"
  Mux/1 -> Gain5/1
  Gain4/1 -> Scope/3
  [w] -> Gain4/1  "w"
  [theta0] -> Mux/1  "theta0"
  [vd] -> Scope/1  "vd"
  Gain5/1 -> Scope/4
  [theta] -> Mux/2  "theta"
  Demux1/1 -> [vd]
  Constant3/1 -> Gain1/1
  Math Function1/1 -> "abc -> dq (Power-Invariant)"/2, [theta], theta/1

== system synchro_v3/PLL Inverter3/PLL (vabc -> vq) ==
  note: Measurement
  note: Gpll
  vabc : Inport
  Constant1 : Constant
  Constant2 : Constant  Value=theta0
  Constant3 : Constant
  Constant4 : Constant  Value=2*pi
  Constant6 : Constant  Value=0
  Demux1 : Demux  Outputs=2
  Discrete PI : SimplexPS/Discrete PI  Kp=w_pll  Ki=w_pll^2/4  xmax=inf  xmin=-inf  Ts=Ts
      settings: SourceProductName=Simplex Power Systems
  Discrete-Time Integrator : DiscreteIntegrator  SampleTime=Ts  ICPrevOutput=DiscIntNeverNeededParam  ICPrevScaledInput=DiscIntNeverNeededParam
  Filter p : DiscreteTransferFcn  Numerator=w_tau*Ts  Denominator=[1 ((w_tau*Ts)-1)]  SampleTime=Ts
  Gain1 : Gain  Gain=Wbase
  Gain2 : Gain  Gain=1/Vbase
  Gain4 : Gain  Gain=1/Wbase
  Gain5 : Gain  Gain=1/pi
  Math Function1 : Math  Operator=mod  SignedPower=on  SaturateOnIntegerOverflow=on
  Mux : Mux  Inputs=2
  Scope : Scope  NumInputPorts=4
  Sum : Sum
  Sum1 : Sum
  "abc -> dq (Power-Invariant)" : SimplexPS/abc -> dq (Power-Invariant)  SystemSampleTime=-1  VariantActivationTime=update diagram  Latency=0  AutoFrameSizeCalculation=off
      settings: SourceProductName=Simplex Power Systems
  w : Outport
  theta : Outport  Port=2
  wires:
  vabc/1 -> "abc -> dq (Power-Invariant)"/1
  "abc -> dq (Power-Invariant)"/1 -> Demux1/1
  Constant4/1 -> Math Function1/2
  Gain2/1 -> Filter p/1
  Demux1/2 -> [vq], Gain2/1
  Constant6/1 -> Discrete PI/4, Discrete PI/3
  Constant1/1 -> Discrete PI/1
  Discrete PI/1 -> Sum/1
  Sum/1 -> [w], w/1, Discrete-Time Integrator/1
  Gain1/1 -> Sum/2
  Discrete-Time Integrator/1 -> Sum1/1
  Sum1/1 -> Math Function1/1
  Constant2/1 -> [theta0], Sum1/2
  Filter p/1 -> Discrete PI/2
  [vq] -> Scope/2  "vq"
  Mux/1 -> Gain5/1
  Gain4/1 -> Scope/3
  [w] -> Gain4/1  "w"
  [theta0] -> Mux/1  "theta0"
  [vd] -> Scope/1  "vd"
  Gain5/1 -> Scope/4
  [theta] -> Mux/2  "theta"
  Demux1/1 -> [vd]
  Constant3/1 -> Gain1/1
  Math Function1/1 -> "abc -> dq (Power-Invariant)"/2, [theta], theta/1

== system synchro_v3/Voltage-Type Inverter (Droop)2/Frequency Droop (iq) ==
  iabc : Inport
  Constant : Constant  Value=W0
  Constant2 : Constant  Value=theta0
  Constant4 : Constant  Value=2*pi
  Constant6 : Constant  Value=P0
  Demux1 : Demux  Outputs=2
  Discrete-Time Integrator : DiscreteIntegrator  SampleTime=Ts  ICPrevOutput=DiscIntNeverNeededParam  ICPrevScaledInput=DiscIntNeverNeededParam
  Filter p : DiscreteTransferFcn  Numerator=w_tau*Ts  Denominator=[1 ((w_tau*Ts)-1)]  SampleTime=Ts
  Gain : Gain  Gain=1/(2*pi)
  Gain1 : Gain  Gain=1/(Sbase/Vbase)
  Gain2 : Gain  Gain=m
  Gain3 : Gain  Gain=Wbase
  Gain4 : Gain  Gain=-1
  Math Function1 : Math  Operator=mod  SignedPower=on  SaturateOnIntegerOverflow=on
  Sum : Sum
  Sum1 : Sum
  Sum2 : Sum  Inputs=+-
  "abc -> dq (Power-Invariant)" : SimplexPS/abc -> dq (Power-Invariant)  SystemSampleTime=-1  VariantActivationTime=update diagram  Latency=0  AutoFrameSizeCalculation=off
      settings: SourceProductName=Simplex Power Systems
  w : Outport
  freq : Outport  Port=2
  theta : Outport  Port=3
  wires:
  Gain4/1 -> Gain1/1
  Demux1/2 -> Gain4/1
  Gain3/1 -> Discrete-Time Integrator/1, Gain/1, w/1
  Sum/1 -> Gain3/1
  Gain/1 -> freq/1
  Sum2/1 -> Gain2/1
  Constant6/1 -> Sum2/1
  iabc/1 -> "abc -> dq (Power-Invariant)"/1
  Constant4/1 -> Math Function1/2
  "abc -> dq (Power-Invariant)"/1 -> Demux1/1
  Constant/1 -> Sum/2
  Gain1/1 -> Filter p/1
  Discrete-Time Integrator/1 -> Sum1/1
  Gain2/1 -> Sum/1
  Math Function1/1 -> "abc -> dq (Power-Invariant)"/2, theta/1
  Constant2/1 -> Sum1/2
  Sum1/1 -> Math Function1/1
  Filter p/1 -> Sum2/2
